simulink library "SaturationCallback"  (Simulink 8.5)
settings: Solver=ode45  StartTime=0.0  StopTime=10.0  RelTol=1e-3
libraries: SaturationCallback x1
settings Model: Creator=moritz  LastModifiedBy=moritz

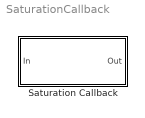
== system SaturationCallback ==
  Saturation Callback : Subsystem  mask{SelectionRadiobutton=Guided, TypePopup=Auto, SubTypePopup=Virtuell, VariantPopup=V9, VariablePopup=GangschaltungMode, ModelVariableEdit=componentManager.Auto.V9.Variables.GangschaltungMode}
      mask prompts: SelectionRadiobutton "Selection Mode"; TypePopup "Type"; SubTypePopup "SubType"; VariantPopup "Variant"; VariablePopup "Variable"; ModelVariableEdit "Model Variable"
      mask init:
      | % Get global variables
      | global componentManager;
      | 
      | % Do nothing if Manual mode is selected
      | selection = get_param(gcb, 'SelectionRadiobutton');
      | if(strcmp(selection, 'Manual'))
      |     path = get_param(gcb, 'ModelVariableEdit');
      |     modelVariable = eval(path);
      |     return;
      | end
      | 
      | % Get mask widgets
      | mask = Simulink.Mask.get(gcb);
      | selection = get_param(gcb, 'SelectionRadiobutton');
      | typePopup = mask.getParameter('TypePopup');
      | subTypePopup = mask.getParameter('SubTypePopup');
      | variantPopup = mask.getParameter('VariantPopup');
      | variablePopup = mask.getParameter('VariablePopup');
      | 
      | % Set Widgets -------------------------------------------------------------
      | % Set type widget
      | types = sort(componentManager.GetTypes());
      | typePopup.set('TypeOptions',types);
      | type = get_param(gcb, 'TypePopup');
      | 
      | % Set subType widget
      | subTypes = sort(componentManager.GetSubTypes(type));
      | if(isempty(subTypes))
      |     subType = '';
      |     subTypePopup.set('Visible', 'off');
      | else
      |     subTypePopup.set('TypeOptions', subTypes);
      |     subTypePopup.set('Visible', 'on');
      |     subType = get_param(gcb, 'SubTypePopup');
      | end
      | 
      | % Set variant widget
      | variants = sort(componentManager.GetVariants(type, subType));
      | variantPopup.set('TypeOptions', variants);
      | variant = get_param(gcb, 'VariantPopup');
      | 
      | % Set variable widget
      | component = componentManager.GetActiveComponent(type, subType, variant);
      | variables = sort(component.GetVariableNames());
      | variablePopup.set('TypeOptions', variables);
      | variable = get_param(gcb, 'VariablePopup');
      | 
      | % Set ModelVariable Edit widget
      | path = componentManager.GetActiveVariablePath(type, subType, variant, variable);
      | set_param(gcb, 'ModelVariableEdit', path);
      mask TypeOptions SelectionRadiobutton: Guided | Manual
      mask Callback SelectionRadiobutton: SaturationCallbackSelection(gcb);
      mask TypeOptions TypePopup: Atm | Auto | Ems | Eq | Gsq | Last | Strecke
      mask Callback TypePopup: modelVariable = SaturationCallbackType(gcb);
      mask TypeOptions SubTypePopup: Real | Virtuell
      mask Callback SubTypePopup:
      | global componentManager;
      | type = get_param(gcb, 'TypePopup');
      | if(componentManager.HasSubType(type))
      |     modelVariable = SaturationCallbackSubType(gcb);
      | end
      | clear type;
      mask TypeOptions VariantPopup: V10 | V8 | V9
      mask Callback VariantPopup: modelVariable = SaturationCallbackVariant(gcb);
      mask TypeOptions VariablePopup: BremsProzentKurveFile | Eta | EtaAchse | EtaGetriebe | Gang1Uebersetzung | Gang2ObereDrehzahl | Gang2Uebersetzung | Gang2UntereDrehzahl | Gang3ObereDrehzahl | Gang3Uebersetzung | Gang3UntereDrehzahl | Gang4ObereDrehzahl | Gang4Uebersetzung | Gang4UntereDrehzahl | Gang5ObereDrehzahl | Gang5Uebersetzung | Gang5UntereDrehzahl | GangschaltungMode | I1 | I2 | J | K | Kupplungsvorgang | Leermasse | MBremsMax | MBremsMaxKurve | MMax | MMaxReal | MMaxStandard | MotorGrenzdrehzahl | Mue0 | MueF | NForM | NForMStandard | Radanzahl | Radradius | RekuperationEnable | Roh | ScaleMode | Schaltverzoegerung | Schwerkraft | SkalierungFest | Stirnflaeche | Stroemungswiderstandskoeffizient | Zuladung
      mask Callback VariablePopup: modelVariable = SaturationCallbackVariable(gcb);

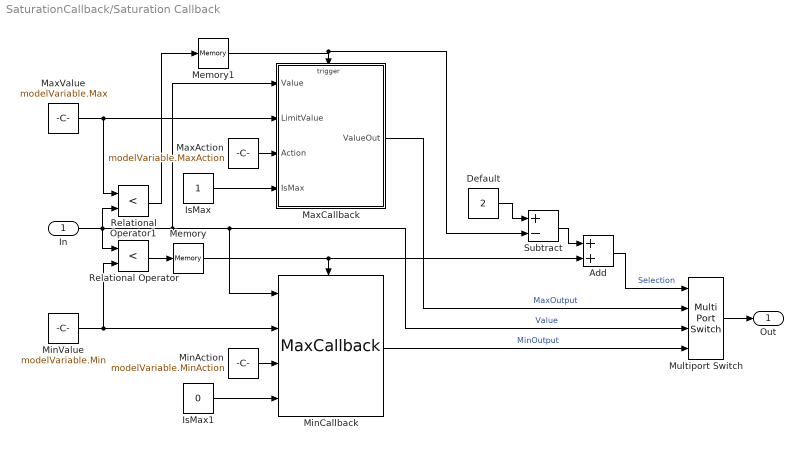
== system SaturationCallback/Saturation Callback ==
  In : Inport
  Add : Sum
  Default : Constant  Value=2
  IsMax : Constant
  IsMax1 : Constant  Value=0
  MaxAction : Constant  Value=modelVariable.MaxAction
  MaxCallback : Subsystem
  MaxValue : Constant  Value=modelVariable.Max
  Memory : Memory
  Memory1 : Memory  InheritSampleTime=on  LinearizeMemory=on
  MinAction : Constant  Value=modelVariable.MinAction
  MinCallback : SaturationCallback/Saturation Callback/MaxCallback
  MinValue : Constant  Value=modelVariable.Min
  Multiport Switch : MultiPortSwitch
  Relational Operator : RelationalOperator  Operator=<  OutDataTypeStr=boolean
  Relational Operator1 : RelationalOperator  Operator=<  OutDataTypeStr=boolean
  Subtract : Sum  Inputs=+-
  Out : Outport
  wires:
  MinValue/1 -> Relational Operator/2, MinCallback/2
  Relational Operator/1 -> Memory/1
  Multiport Switch/1 -> Out/1
  MaxValue/1 -> Relational Operator1/1, MaxCallback/2(LimitValue)
  Relational Operator1/1 -> Memory1/1
  Default/1 -> Subtract/1
  Subtract/1 -> Add/1
  Add/1 -> Multiport Switch/1  "Selection"
  MinAction/1 -> MinCallback/3
  MinCallback/1 -> Multiport Switch/4  "MinOutput"
  MaxCallback/1(ValueOut) -> Multiport Switch/2  "MaxOutput"
  IsMax/1 -> MaxCallback/4(IsMax)
  In/1 -> MaxCallback/1(Value), MinCallback/1, Multiport Switch/3, Relational Operator1/2, Relational Operator/1  "Value"
  IsMax1/1 -> MinCallback/4
  MaxAction/1 -> MaxCallback/3(Action)
  Memory/1 -> MinCallback/Trigger, Add/2
  Memory1/1 -> MaxCallback/Trigger, Subtract/2

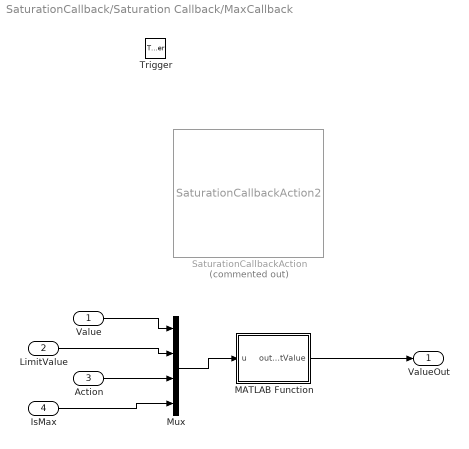
== system SaturationCallback/Saturation Callback/MaxCallback ==
  Value : Inport
  LimitValue : Inport  Port=2
  Action : Inport  Port=3
  IsMax : Inport  Port=4
  Trigger : TriggerPort  PortDimensions=1
  MATLAB Function : MATLAB Function  TreatAsAtomicUnit=on
  Mux : Mux
  SaturationCallbackAction : M-S-Function  Commented=on  FunctionName=SaturationCallbackAction2
  ValueOut : Outport
  wires:
  Action/1 -> Mux/3
  Value/1 -> Mux/1
  LimitValue/1 -> Mux/2
  IsMax/1 -> Mux/4
  Mux/1 -> MATLAB Function/1(u)
  MATLAB Function/1(outputValue) -> ValueOut/1

== matlab function Saturation Callback/MaxCallback/MATLAB Function ==
  data: u input double; outputValue output double
function outputValue = fcn(u)

inputValue = u(1);
limitValue = u(2);
action = u(3);
isMax = u(4);

switch action
    case 1
        fprintf('%s%i%i%i', 'Jo! Prob:', int32(inputValue), int32(limitValue), int32(isMax))
        outputValue = inputValue;
    case 2
        outputValue = limitValue;
        fprintf('%s%i%i%i', 'Jo! Real Prob:', int32(inputValue), int32(limitValue), int32(isMax))
    case 3
        error('Mos:Sat', 'Jo! Shit hit fan:%i, %i, %i', int32(inputValue), int32(limitValue), int32(isMax))
    otherwise
        fprintf('%s%i%i%i', 'No Prob. But here the facts:', int32(inputValue), int32(limitValue), int32(isMax))
        outputValue = inputValue;
end

end
